simulink model "Active_suspension_open_loop"  (R2022b)
settings: Solver=ode1  StartTime=0.0  StopTime=inf  FixedStep=0.001  RelTol=1e-3  EnableMultiTasking=on
values from neighbouring files (symbols this model uses):
  A = [ 0 1 0 -1 ... (first row only)    [Active_suspension_open_loop_setup.m]
  B = [0  0 ; 0 1/ms ; -1  0 ; bus/mu -1/mu ]    [Active_suspension_open_loop_setup.m]
  C = [ 1 0 0 0 ; -ks/ms -bs/ms 0 bs/ms ]    [Active_suspension_open_loop_setup.m]
  D = zeros(6,2); D(6,2)=1/ms    [Active_suspension_open_loop_setup.m]
  K = lqr( A, B(:,2), Q, R )    [Active_suspension_open_loop_setup.m]
settings Model: SimulationMode=external  ExtModeTrigDuration=50000  Creator=DCrymble  LastModifiedBy=admin
settings SolverCC: AlgebraicLoopSolver=TrustRegion  PositivePriorityOrder=on
settings DataIOCC: LimitDataPoints=on  SaveFormat=Array  SignalLoggingSaveFormat=ModelDataLogs  ReturnWorkspaceOutputs=off
settings OptimizationCC: BooleanDataType=off  OptimizeBlockIOStorage=off  BufferReuse=off  GlobalBufferReuse=off  ExpressionFolding=off  ExpressionDepthLimit=2147483647  LocalBlockOutputs=off  InitFltsAndDblsToZero=on  LifeSpan=inf
settings DebuggingCC: UnderspecifiedInitializationDetection=Classic  MergeDetectMultiDrivingBlocksExec=none  SolverPrmCheckMsg=warning  FcnCallInpInsideContextMsg=warning  UnconnectedInputMsg=warning  UnconnectedOutputMsg=warning  UnconnectedLineMsg=warning  StateNameClashWarn=warning  SFUnexpectedBacktrackingDiag=warning  SFNoUnconditionalDefaultTransitionDiag=warning  SFMachineParentedDataDiag=warning  ArithmeticOperatorsInVariantConditions=warning
settings HardwareCC: ProdBitPerPointer=32  ProdBitPerSizeT=32  ProdBitPerPtrDiffT=32  ProdLargestAtomicFloat=None  ProdIntDivRoundTo=Undefined  ProdEndianess=Unspecified  ProdWordSize=32  ProdHWDeviceType=32-bit Generic
settings ModelReferenceCC: EnableRefExpFcnMdlSchedulingChecks=on  PropagateSignalLabelsOutOfModel=off
settings SFSimCC: SimUseLocalCustomCode=off  SimParseCustomCode=off  CustomCodeUndefinedFunction=UseInterfaceOnly
settings RTWCC: Description=QuaRC Win32 Target  SystemTargetFile=quarc_windows.tlc  TemplateMakefile=quarc_default_tmf  RTWUseLocalCustomCode=off
settings CodeAppCC: StateflowObjectComments=on
settings STFCustomTargetCC: TargetPreCompLibLocation=C:\PROGRA~3\QUARC\lib\2016a\windows\release  CPPClassGenCompliant=on  GRTInterface=on  SystemTargetFile=quarc_windows.tlc
settings GRTTargetCC: TargetPreCompLibLocation=C:\PROGRA~3\QUARC\lib\2016a\windows\release  TargetLangStandard=C89/C90 (ANSI)  ParMdlRefBuildCompliant=off  CompOptLevelCompliant=off  ConcurrentExecutionCompliant=off  CombineOutputUpdateFcns=off  MatFileLogging=off  GRTInterface=on  UseToolchainInfoCompliant=off  ExtMode=on  ExtModeMexFile=quarc_comm
settings ConfigComp: CovMetricSettings=dw  CovSaveCumulativeToWorkspaceVar=on  CovSaveSingleToWorkspaceVar=on  CovExternalEMLEnable=off

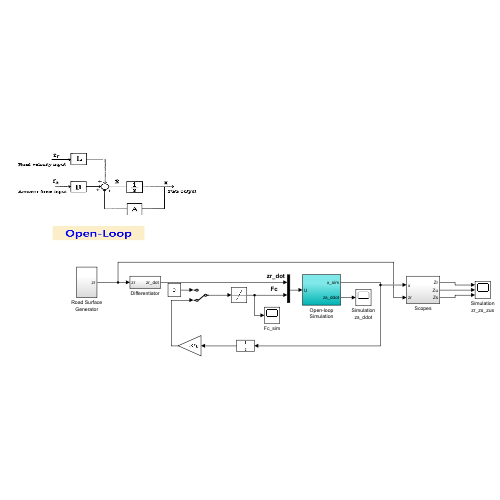
[thumbnail: Simulink's stored preview of the top-level diagram]
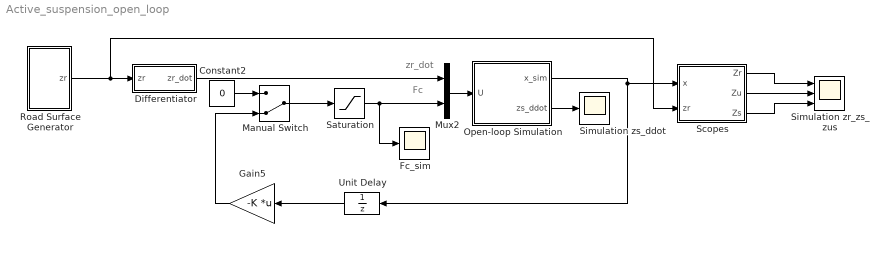
== system Active_suspension_open_loop ==
  note: zr_dot
  note: Fc
  Constant2 : Constant  Value=0
  Differentiator : Subsystem
  Fc_sim : Scope
  Gain5 : Gain  Gain=-K  Multiplication=Matrix(K*u)
  Manual Switch : ManualSwitch  CurrentSetting=0
  Mux2 : Mux  Inputs=2
  Open-loop Simulation : Subsystem
  Road Surface Generator : Subsystem
  Saturation : Saturate  UpperLimit=38.3  LowerLimit=-38.3
  Scopes : Subsystem
  Simulation zr_zs_zus : Scope  NumInputPorts=3
  Simulation zs_ddot : Scope
  Unit Delay : UnitDelay  SampleTime=-1  HasFrameUpgradeWarning=on
  wires:
  Differentiator/1(zr_dot) -> Mux2/1
  Constant2/1 -> Manual Switch/1
  Manual Switch/1 -> Saturation/1
  Mux2/1 -> Open-loop Simulation/1(U)
  Saturation/1 -> Mux2/2, Fc_sim/1
  Gain5/1 -> Manual Switch/2
  Open-loop Simulation/1(x_sim) -> Unit Delay/1, Scopes/1(x)
  Unit Delay/1 -> Gain5/1
  Road Surface Generator/1(zr) -> Scopes/2(zr), Differentiator/1(zr)
  Open-loop Simulation/2(zs_ddot) -> Simulation zs_ddot/1
  Scopes/1(Zr) -> Simulation zr_zs_zus/1
  Scopes/2(Zu) -> Simulation zr_zs_zus/2
  Scopes/3(Zs) -> Simulation zr_zs_zus/3

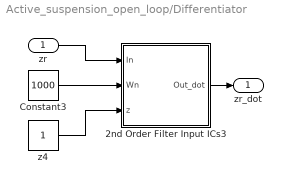
== system Active_suspension_open_loop/Differentiator ==
  zr : Inport
  2nd Order Filter Input ICs3 : Subsystem
  Constant3 : Constant  Value=1000
  z4 : Constant
  zr_dot : Outport
  wires:
  Constant3/1 -> 2nd Order Filter Input ICs3/2(Wn)
  z4/1 -> 2nd Order Filter Input ICs3/3(z)
  zr/1 -> 2nd Order Filter Input ICs3/1(In)
  2nd Order Filter Input ICs3/1(Out_dot) -> zr_dot/1

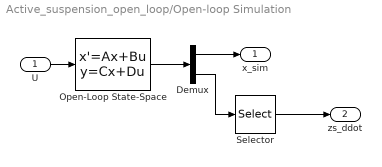
== system Active_suspension_open_loop/Open-loop Simulation ==
  U : Inport
  Demux : Demux  Outputs=[4 2]
  Open-Loop State-Space : StateSpace  A=A  B=B  C=cat(1,eye(4), C)  D=D  InitialCondition=0
  Selector : Selector  InputPortWidth=2  IndexOptions=Index vector (dialog)  Indices=[2]  OutputSizes=1
  x_sim : Outport
  zs_ddot : Outport  Port=2
  wires:
  Open-Loop State-Space/1 -> Demux/1
  Demux/1 -> x_sim/1
  U/1 -> Open-Loop State-Space/1
  Demux/2 -> Selector/1
  Selector/1 -> zs_ddot/1

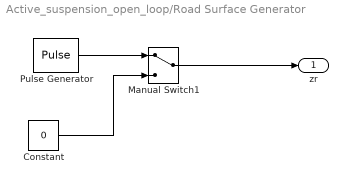
== system Active_suspension_open_loop/Road Surface Generator ==
  Constant : Constant  Value=0
  Manual Switch1 : ManualSwitch
  Pulse Generator : DiscretePulseGenerator  PulseType=Time based  Amplitude=0.02  Period=3  PulseWidth=50  PhaseDelay=.1
  zr : Outport
  wires:
  Constant/1 -> Manual Switch1/2
  Pulse Generator/1 -> Manual Switch1/1
  Manual Switch1/1 -> zr/1

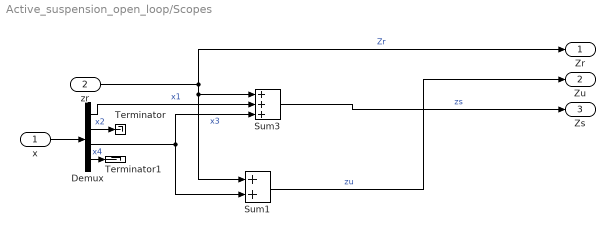
== system Active_suspension_open_loop/Scopes ==
  x : Inport
  zr : Inport  Port=2
  Demux : Demux
  Sum1 : Sum  Inputs=2  InputSameDT=on  SaturateOnIntegerOverflow=on  OutDataTypeStr=Inherit: Same as first input
  Sum3 : Sum  Inputs=3  InputSameDT=on  SaturateOnIntegerOverflow=on  OutDataTypeStr=Inherit: Same as first input
  Terminator : Terminator
  Terminator1 : Terminator
  Zr : Outport
  Zu : Outport  Port=2
  Zs : Outport  Port=3
  wires:
  Demux/1 -> Sum3/2  "x1"
  Demux/3 -> Sum3/3, Sum1/2  "x3"
  zr/1 -> Zr/1, Sum3/1, Sum1/1  "Zr"
  x/1 -> Demux/1
  Sum1/1 -> Zu/1  "zu"
  Sum3/1 -> Zs/1  "zs"
  Demux/2 -> Terminator/1  "x2"
  Demux/4 -> Terminator1/1  "x4"

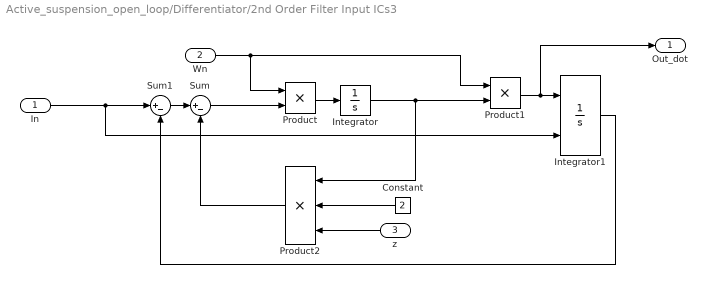
== system Active_suspension_open_loop/Differentiator/2nd Order Filter Input ICs3 ==
  In : Inport
  Wn : Inport  Port=2
  z : Inport  Port=3
  Constant : Constant  Value=2
  Integrator : Integrator
  Integrator1 : Integrator  InitialConditionSource=external
  Product : Product  RndMeth=Zero
  Product1 : Product  RndMeth=Zero
  Product2 : Product  Inputs=3  RndMeth=Zero
  Sum : Sum  Inputs=|+-
  Sum1 : Sum  Inputs=|+-
  Out_dot : Outport
  wires:
  Constant/1 -> Product2/2
  z/1 -> Product2/3
  Product2/1 -> Sum/2
  In/1 -> Integrator1/2, Sum1/1
  Sum1/1 -> Sum/1
  Integrator1/1 -> Sum1/2
  Integrator/1 -> Product2/1, Product1/2
  Product1/1 -> Out_dot/1, Integrator1/1
  Wn/1 -> Product1/1, Product/1
  Sum/1 -> Product/2
  Product/1 -> Integrator/1
